simulink model "cruise_Control_Model"  (R2020a)
settings: Solver=VariableStepAuto  StartTime=0.0  StopTime=10.0  RelTol=1e-3
undefined symbols (not defined in the file or in its folder): Kd, Ki, Kp
settings Model: Creator=INDRAJIT MARATHE  LastModifiedBy=INDRAJIT MARATHE

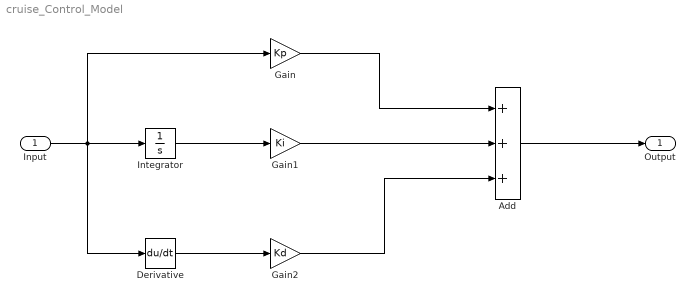
== system cruise_Control_Model ==
  Input : Inport
  Add : Sum  Inputs=+++
  Derivative : Derivative
  Gain : Gain  Gain=Kp
  Gain1 : Gain  Gain=Ki
  Gain2 : Gain  Gain=Kd
  Integrator : Integrator
  Output : Outport
  wires:
  Gain1/1 -> Add/2
  Gain2/1 -> Add/3
  Gain/1 -> Add/1
  Integrator/1 -> Gain1/1
  Derivative/1 -> Gain2/1
  Input/1 -> Derivative/1, Gain/1, Integrator/1
  Add/1 -> Output/1
